simulink library "Triad_lib"  (R2018b)
settings: Solver=VariableStepAuto  StartTime=0.0  StopTime=10.0  RelTol=1e-3
undefined symbols (not defined in the file): fswParams
libraries: vrlib x6, dspmathops x2, parallel_protection_lib x2, sharedutil x1, sharedtransform x1
settings Model: Creator=kylle  LastModifiedBy=Taylor

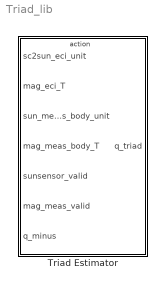
== system Triad_lib ==
  Triad Estimator : Subsystem  TreatAsAtomicUnit=on

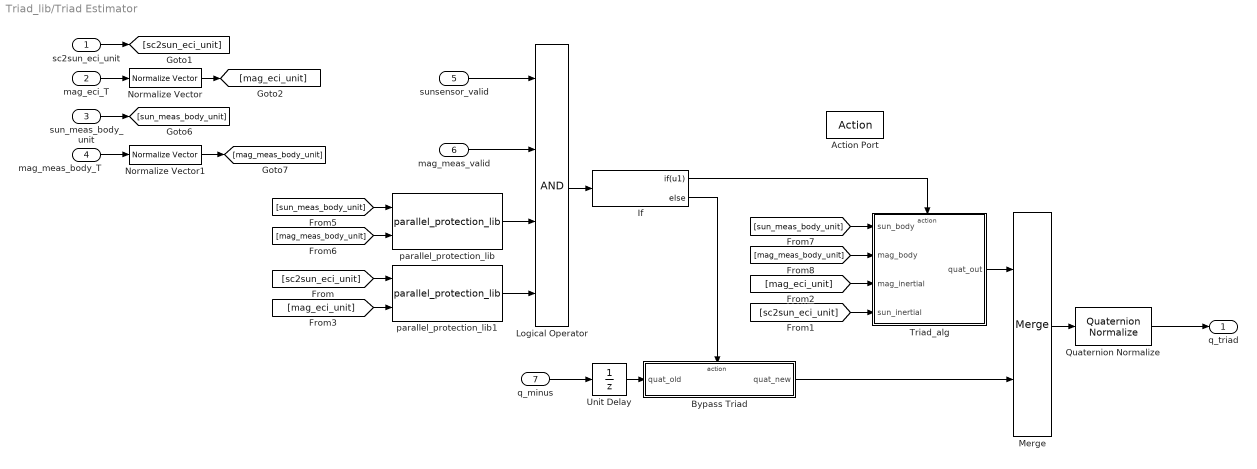
== system Triad_lib/Triad Estimator ==
  sc2sun_eci_unit : Inport
  mag_eci_T : Inport  Port=2
  sun_meas_body_unit : Inport  Port=3
  mag_meas_body_T : Inport  Port=4
  sunsensor_valid : Inport  Port=5
  mag_meas_valid : Inport  Port=6
  q_minus : Inport  Port=7
  Action Port : ActionPort
  Bypass Triad : Subsystem  TreatAsAtomicUnit=on
  If : If  IfExpression=u1
  Logical Operator : Logic  Inputs=4  AllPortsSameDT=off  OutDataTypeStr=boolean
  Merge : Merge
  Normalize Vector : vrlib/Utilities/Normalize Vector  maxzero=0
      settings: SourceProductName=Simulink 3D Animation  SourceProductBaseCode=VR
  Normalize Vector1 : vrlib/Utilities/Normalize Vector  maxzero=0
      settings: SourceProductName=Simulink 3D Animation  SourceProductBaseCode=VR
  Quaternion Normalize : sharedutil/Quaternion Normalize  aMode=aMode
      settings: SourceProductName=Aerospace Blockset  SourceProductBaseCode=AE
  Triad_alg : Subsystem  TreatAsAtomicUnit=on
  Unit Delay : UnitDelay  InitialCondition=fswParams.estimation.ic.quat_est_init  SampleTime=fswParams.sample_time_s
  parallel_protection_lib : parallel_protection_lib/parallel_protection_lib  min_angle_deg=fswParams.estimation.triad_parallel_tol_deg
  parallel_protection_lib1 : parallel_protection_lib/parallel_protection_lib  min_angle_deg=fswParams.estimation.triad_parallel_tol_deg
  q_triad : Outport
  wires:
  Merge/1 -> Quaternion Normalize/1
  If/1 -> Triad_alg/Action
  If/2 -> Bypass Triad/Action
  Triad_alg/1(quat_out) -> Merge/1
  Bypass Triad/1(quat_new) -> Merge/2
  Logical Operator/1 -> If/1
  Quaternion Normalize/1 -> q_triad/1
  Unit Delay/1 -> Bypass Triad/1(quat_old)
  parallel_protection_lib/1 -> Logical Operator/3
  [sun_meas_body_unit] -> Triad_alg/1(sun_body)
  [mag_meas_body_unit] -> Triad_alg/2(mag_body)
  sunsensor_valid/1 -> Logical Operator/1
  mag_meas_valid/1 -> Logical Operator/2
  sun_meas_body_unit/1 -> [sun_meas_body_unit]
  [sun_meas_body_unit] -> parallel_protection_lib/1
  mag_meas_body_T/1 -> Normalize Vector1/1
  [mag_meas_body_unit] -> parallel_protection_lib/2
  sc2sun_eci_unit/1 -> [sc2sun_eci_unit]
  [sc2sun_eci_unit] -> Triad_alg/4(sun_inertial)
  [mag_eci_unit] -> Triad_alg/3("mag_inertial ")
  mag_eci_T/1 -> Normalize Vector/1
  Normalize Vector/1 -> [mag_eci_unit]
  Normalize Vector1/1 -> [mag_meas_body_unit]
  parallel_protection_lib1/1 -> Logical Operator/4
  [mag_eci_unit] -> parallel_protection_lib1/2
  [sc2sun_eci_unit] -> parallel_protection_lib1/1
  q_minus/1 -> Unit Delay/1

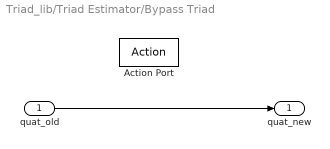
== system Triad_lib/Triad Estimator/Bypass Triad ==
  quat_old : Inport
  Action Port : ActionPort
  quat_new : Outport
  wires:
  quat_old/1 -> quat_new/1

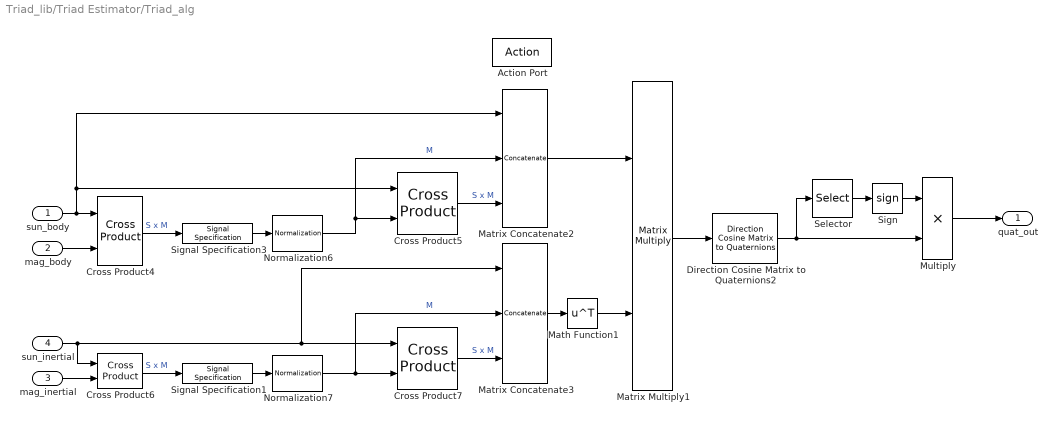
== system Triad_lib/Triad Estimator/Triad_alg ==
  sun_body : Inport
  mag_body : Inport  Port=2
  "mag_inertial " : Inport  Port=3
  sun_inertial : Inport  Port=4
  Action Port : ActionPort
  Cross Product{4..7} (4 alike) : vrlib/Utilities/Cross Product
      settings: SourceProductBaseCode=VR
  Direction Cosine Matrix to Quaternions2 : sharedtransform/Direction Cosine Matrix  to Quaternions  aMode=0  action=None  tolerance=eps(2)
      settings: SourceProductName=Aerospace Blockset  SourceProductBaseCode=AE
  Math Function1 : Math  Operator=transpose  SaturateOnIntegerOverflow=on
  Matrix Concatenate2 : Concatenate  NumInputs=3  Mode=Multidimensional array  ConcatenateDimension=2
  Matrix Concatenate3 : Concatenate  NumInputs=3  Mode=Multidimensional array  ConcatenateDimension=2
  Matrix Multiply1 : Product  Multiplication=Matrix(*)
  Multiply : Product
  Normalization6 : dspmathops/Normalization  NormType=2-norm  Bias=1e-10  NormOver=Each column  Dimension=1  roundingMode=Floor  overflowMode=off  accumDataTypeStr=Inherit: Same as product output  accumLastDataTypeStr=Inherit: Same as product output  outputDataTypeStr=Inherit: Same as product output  outputMin=[]  outputMax=[]  outputLastDataTypeStr=Inherit: Same as product output
      settings: SourceProductName=DSP System Toolbox
  Normalization7 : dspmathops/Normalization  NormType=2-norm  Bias=1e-10  NormOver=Each column  Dimension=1  roundingMode=Floor  overflowMode=off  accumDataTypeStr=Inherit: Same as product output  accumLastDataTypeStr=Inherit: Same as product output  outputDataTypeStr=Inherit: Same as product output  outputMin=[]  outputMax=[]  outputLastDataTypeStr=Inherit: Same as product output
      settings: SourceProductName=DSP System Toolbox
  Selector : Selector  InputPortWidth=4  IndexOptions=Index vector (dialog)  Indices=[1]  OutputSizes=1
  Sign : Signum
  Signal Specification1 : SignalSpecification  Dimensions=3
  Signal Specification3 : SignalSpecification  Dimensions=3
  quat_out : Outport
  wires:
  Signal Specification3/1 -> Normalization6/1
  sun_body/1 -> Matrix Concatenate2/1, Cross Product5/1, Cross Product4/1
  mag_body/1 -> Cross Product4/2
  Cross Product4/1 -> Signal Specification3/1  "S x M"
  Normalization6/1 -> Matrix Concatenate2/2, Cross Product5/2  "M"
  Cross Product5/1 -> Matrix Concatenate2/3  "S x M"
  sun_inertial/1 -> Cross Product6/1, Matrix Concatenate3/1, Cross Product7/1
  Cross Product7/1 -> Matrix Concatenate3/3  "S x M"
  Normalization7/1 -> Matrix Concatenate3/2, Cross Product7/2  "M"
  Cross Product6/1 -> Signal Specification1/1  "S x M"
  "mag_inertial "/1 -> Cross Product6/2
  Matrix Concatenate3/1 -> Math Function1/1
  Matrix Multiply1/1 -> Direction Cosine Matrix to Quaternions2/1
  Matrix Concatenate2/1 -> Matrix Multiply1/1
  Math Function1/1 -> Matrix Multiply1/2
  Direction Cosine Matrix to Quaternions2/1 -> Multiply/2, Selector/1
  Sign/1 -> Multiply/1
  Selector/1 -> Sign/1
  Multiply/1 -> quat_out/1
  Signal Specification1/1 -> Normalization7/1
